simulink model "ModeleCompletSimple"  (R2019b)
settings: Solver=VariableStepAuto  StartTime=0.0  StopTime=10  RelTol=1e-3
libraries: dspsrcs4 x1
settings Model: Creator=jeanz  LastModifiedBy=maxim

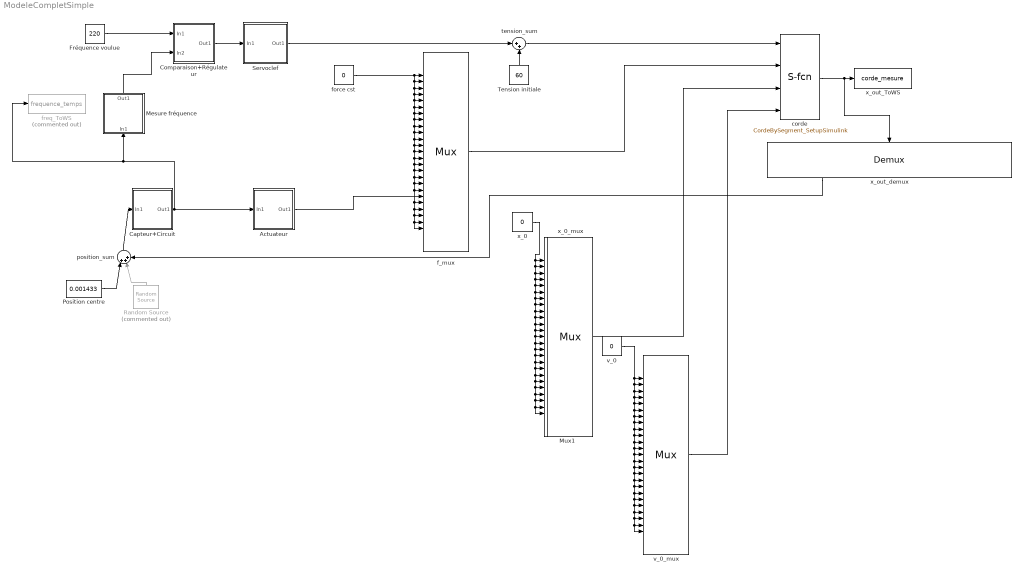
== system ModeleCompletSimple ==
  Actuateur : Subsystem
  Capteur+Circuit : Subsystem
  Comparaison+Régulateur : Subsystem
  Fréquence voulue : Constant  Value=220
  Mesure fréquence : Subsystem
  Mux1 : Mux  Inputs=25
      settings: DisplayOption=signals
  Position centre : Constant  Value=0.001433
  Random Source : dspsrcs4/Random Source  Commented=on  SrcType=Uniform  NormMethod=Ziggurat  CltLength=12  MinVal=-0.0001  MaxVal=0.0001  MeanVal=0  VarVal=1  RepMode=Not repeatable  rawSeed=1  IsInherit=off  SampMode=Discrete  SampTime=1  SampFrame=1  DataType=Double  OutComplex=Real  OutputFrames=off
  Servoclef : Subsystem
  Tension initiale : Constant  Value=60
  corde : M-S-Function  FunctionName=CordeBySegment_SetupSimulink  Parameters=0.00325, 0.44, 0.0326, 25, 0.001
  f_mux : Mux  Inputs=25
  force cst : Constant  Value=0
  freq_ToWS : ToWorkspace  Commented=on  VariableName=frequence_temps  SaveFormat=Timeseries  SampleTime=0.0005
  position_sum : Sum  Inputs=|+++
  tension_sum : Sum  Inputs=|++
  v_0 : Constant  Value=0
  v_0_mux : Mux  Inputs=25
  x_0 : Constant  Value=0
  x_0_mux : Mux  Inputs=25
  x_out_ToWS : ToWorkspace  VariableName=corde_mesure  SaveFormat=Timeseries  SampleTime=0.0005
  x_out_demux : Demux  Outputs=25
  wires:
  v_0_mux/1 -> corde/4
  x_0/1 -> Mux1/1, Mux1/2, Mux1/3, Mux1/4, Mux1/6, Mux1/12, Mux1/20, Mux1/25, Mux1/24, Mux1/23, Mux1/22, Mux1/21, Mux1/19, Mux1/18, Mux1/17, Mux1/16, Mux1/15, Mux1/14, Mux1/13, Mux1/11, Mux1/10, Mux1/9, Mux1/8, Mux1/7, Mux1/5
  v_0/1 -> v_0_mux/1, v_0_mux/2, v_0_mux/3, v_0_mux/4, v_0_mux/6, v_0_mux/25, v_0_mux/24, v_0_mux/23, v_0_mux/22, v_0_mux/21, v_0_mux/20, v_0_mux/19, v_0_mux/18, v_0_mux/17, v_0_mux/16, v_0_mux/15, v_0_mux/14, v_0_mux/13, v_0_mux/12, v_0_mux/11, v_0_mux/10, v_0_mux/9, v_0_mux/8, v_0_mux/7, v_0_mux/5
  f_mux/1 -> corde/2
  Mux1/1 -> corde/3
  force cst/1 -> f_mux/18, f_mux/25, f_mux/24, f_mux/23, f_mux/22, f_mux/21, f_mux/19, f_mux/17, f_mux/16, f_mux/15, f_mux/14, f_mux/13, f_mux/12, f_mux/11, f_mux/10, f_mux/9, f_mux/8, f_mux/7, f_mux/6, f_mux/5, f_mux/4, f_mux/3, f_mux/2, f_mux/1
  corde/1 -> x_out_demux/1, x_out_ToWS/1
  Comparaison+Régulateur/1(Out1) -> Servoclef/1(In1)
  Actuateur/1(Out1) -> f_mux/20
  Mesure fréquence/1(Out1) -> Comparaison+Régulateur/2(In2)
  Fréquence voulue/1 -> Comparaison+Régulateur/1(In1)
  position_sum/1 -> Capteur+Circuit/1(In1)
  Position centre/1 -> position_sum/1
  Tension initiale/1 -> tension_sum/2
  Servoclef/1(Out1) -> tension_sum/1
  tension_sum/1 -> corde/1
  Capteur+Circuit/1(Out1) -> freq_ToWS/1, Mesure fréquence/1(In1), Actuateur/1(In1)
  Random Source/1 -> position_sum/2
  x_out_demux/6 -> position_sum/3

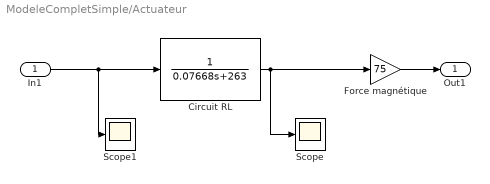
== system ModeleCompletSimple/Actuateur ==
  In1 : Inport
  Circuit RL : TransferFcn  Denominator=[0.07668 263]
  Force magnétique : Gain  Gain=75
  Scope : Scope
  Scope1 : Scope
  Out1 : Outport
  wires:
  Force magnétique/1 -> Out1/1
  Circuit RL/1 -> Force magnétique/1, Scope/1
  In1/1 -> Scope1/1, Circuit RL/1

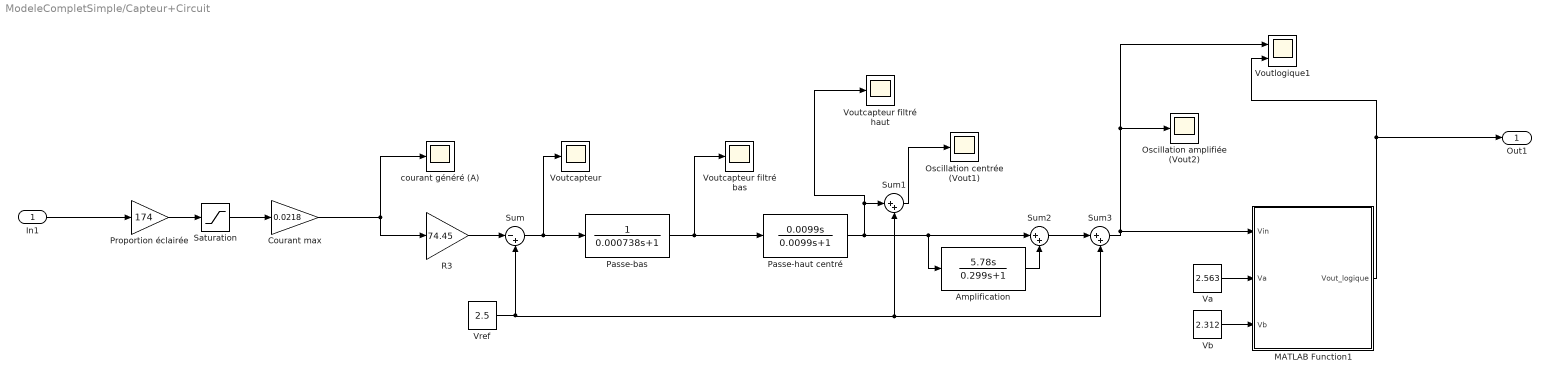
== system ModeleCompletSimple/Capteur+Circuit ==
  In1 : Inport
  "Amplification " : TransferFcn  Numerator=[5.78 0]  Denominator=[0.299 1]
  Courant max : Gain  Gain=0.0218
  MATLAB Function1 : MATLAB Function  TreatAsAtomicUnit=on
  "Oscillation amplifiée (Vout2) " : Scope
  Oscillation centrée (Vout1) : Scope
  Passe-bas : TransferFcn  Denominator=[0.000738 1]
  "Passe-haut centré " : TransferFcn  Numerator=[0.0099 0]  Denominator=[0.0099 1]
  Proportion éclairée : Gain  Gain=174
  R3 : Gain  Gain=74.45
  Saturation : Saturate  UpperLimit=0.497  LowerLimit=0
  Sum : Sum  Inputs=|-+
  Sum1 : Sum  Inputs=|++
  Sum2 : Sum  Inputs=|++
  Sum3 : Sum  Inputs=|++
  "Va " : Constant  Value=2.563
  Vb : Constant  Value=2.312
  "Voutcapteur " : Scope
  Voutcapteur filtré bas : Scope
  Voutcapteur filtré haut : Scope
  Voutlogique1 : Scope  NumInputPorts=2
  "Vref " : Constant  Value=2.5
  "courant généré (A) " : Scope
  Out1 : Outport
  wires:
  "Amplification "/1 -> Sum2/2
  Sum3/1 -> Voutlogique1/1, "Oscillation amplifiée (Vout2) "/1, MATLAB Function1/1(Vin)
  "Vref "/1 -> Sum/2, Sum3/2, Sum1/2
  Sum/1 -> "Voutcapteur "/1, Passe-bas/1
  R3/1 -> Sum/1
  "Passe-haut centré "/1 -> Sum2/1, "Amplification "/1, Voutcapteur filtré haut/1, Sum1/1
  Vb/1 -> MATLAB Function1/3(Vb)
  Passe-bas/1 -> Voutcapteur filtré bas/1, "Passe-haut centré "/1
  Sum2/1 -> Sum3/1
  Sum1/1 -> Oscillation centrée (Vout1)/1
  MATLAB Function1/1(Vout_logique) -> Out1/1, Voutlogique1/2
  "Va "/1 -> MATLAB Function1/2(Va)
  Saturation/1 -> Courant max/1
  Proportion éclairée/1 -> Saturation/1
  Courant max/1 -> R3/1, "courant généré (A) "/1
  In1/1 -> Proportion éclairée/1

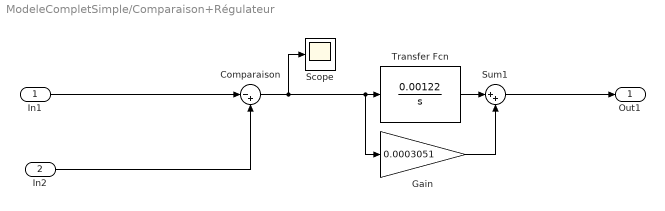
== system ModeleCompletSimple/Comparaison+Régulateur ==
  In1 : Inport
  In2 : Inport  Port=2
  Comparaison : Sum  Inputs=|-+
  Gain : Gain  Gain=0.0003051
  Scope : Scope
  Sum1 : Sum  Inputs=|++
  Transfer Fcn : TransferFcn  Numerator=[0.00122]  Denominator=[1 0]
  Out1 : Outport
  wires:
  Comparaison/1 -> Scope/1, Gain/1, Transfer Fcn/1
  In1/1 -> Comparaison/1
  Transfer Fcn/1 -> Sum1/1
  Gain/1 -> Sum1/2
  Sum1/1 -> Out1/1
  In2/1 -> Comparaison/2

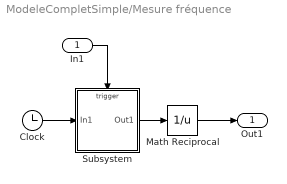
== system ModeleCompletSimple/Mesure fréquence ==
  In1 : Inport
  Clock : Clock
  Math Reciprocal : Math  Operator=reciprocal  SaturateOnIntegerOverflow=on
  Subsystem : Subsystem
  Out1 : Outport
  wires:
  In1/1 -> Subsystem/Trigger
  Clock/1 -> Subsystem/1(In1)
  Math Reciprocal/1 -> Out1/1
  Subsystem/1(Out1) -> Math Reciprocal/1

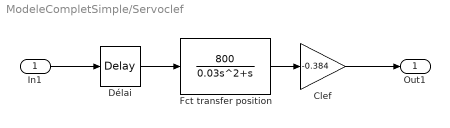
== system ModeleCompletSimple/Servoclef ==
  In1 : Inport
  Clef : Gain  Gain=-0.384
  Délai : TransportDelay  DelayTime=0.01
  Fct transfer position : TransferFcn  Numerator=[800]  Denominator=[0.03 1 0]
  Out1 : Outport
  wires:
  Fct transfer position/1 -> Clef/1
  Clef/1 -> Out1/1
  Délai/1 -> Fct transfer position/1
  In1/1 -> Délai/1

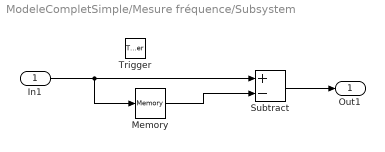
== system ModeleCompletSimple/Mesure fréquence/Subsystem ==
  In1 : Inport
  Trigger : TriggerPort  VariantControl=Variant  PortDimensions=1
  Memory : Memory  InheritSampleTime=on
  Subtract : Sum  Inputs=+-
  Out1 : Outport
  wires:
  In1/1 -> Memory/1, Subtract/1
  Memory/1 -> Subtract/2
  Subtract/1 -> Out1/1

== matlab function ModeleCompletSimple/Capteur+Circuit/MATLAB Function1 ==
  data: Vin input; Vout_logique output; Va input; Vb input
function Vout_logique = fcn(Vin, Va, Vb)

Vout_logique = 0;
if Vin > Va && Vout_logique == 5
    Vout_logique = 0;
end
if Vin < Vb && Vout_logique == 0
    Vout_logique = 5;
end
end
